simulink model "CBF_for_DoubleInteg"  (R2024a)
settings: Solver=VariableStepAuto  StartTime=0.0  StopTime=Tf  RelTol=1e-3
undefined symbols (not defined in the file): M, Ts, x1_0, x2_0
libraries: slctrl_constraint x1
settings Model: Creator=bumyong  LastModifiedBy=bumyong

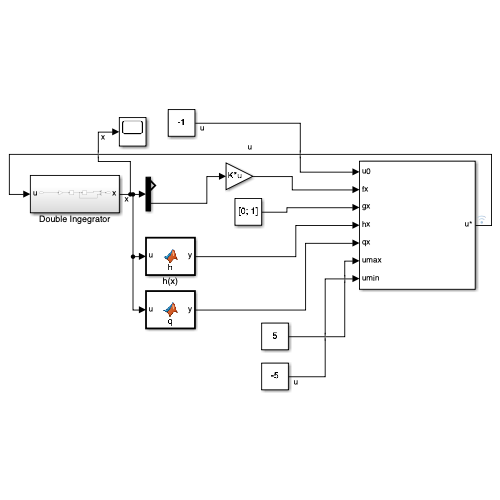
[thumbnail: Simulink's stored preview of the top-level diagram]
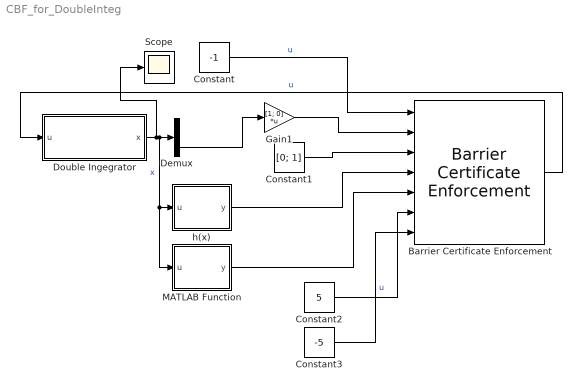
== system CBF_for_DoubleInteg ==
  Barrier Certificate Enforcement : slctrl_constraint/Barrier Certificate Enforcement  nx=2  nu=1  nc=4  gamma=gamma  beta=1  external_umax=on  external_umin=on  Ts=Ts  maxiter=200  tol=1e-6  output_exitflag=on
      settings: LibrarySourceBlock=slctrlblks/Constraint Control/Barrier Certificate Enforcement
  Constant : Constant  Value=-1
  Constant1 : Constant  Value=[0; 1]
  Constant2 : Constant  Value=5
  Constant3 : Constant  Value=-5
  Demux : Demux  Outputs=2
  Double Ingegrator : Subsystem
  Gain1 : Gain  Gain=[1; 0]  Multiplication=Matrix(K*u)
  MATLAB Function : MATLAB Function  TreatAsAtomicUnit=on
  Scope : Scope
  h(x) : MATLAB Function  TreatAsAtomicUnit=on
  wires:
  Constant/1 -> Barrier Certificate Enforcement/1  "u"
  Barrier Certificate Enforcement/1 -> Double Ingegrator/1(u)  "u"
  Constant1/1 -> Barrier Certificate Enforcement/3
  Double Ingegrator/1(x) -> Scope/1, MATLAB Function/1(u), h(x)/1(u), Demux/1  "x"
  Demux/2 -> Gain1/1
  Gain1/1 -> Barrier Certificate Enforcement/2
  h(x)/1(y) -> Barrier Certificate Enforcement/4
  MATLAB Function/1(y) -> Barrier Certificate Enforcement/5
  Constant2/1 -> Barrier Certificate Enforcement/6
  Constant3/1 -> Barrier Certificate Enforcement/7  "u"

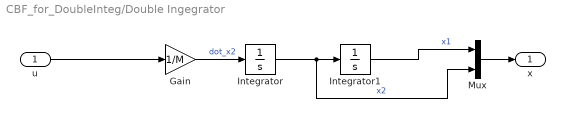
== system CBF_for_DoubleInteg/Double Ingegrator ==
  u : Inport
  Gain : Gain  Gain=1/M
  Integrator : Integrator  InitialCondition=x2_0
  Integrator1 : Integrator  InitialCondition=x1_0
  Mux : Mux  Inputs=2
  x : Outport
  wires:
  Gain/1 -> Integrator/1  "dot_x2"
  Integrator/1 -> Mux/2, Integrator1/1  "x2"
  u/1 -> Gain/1
  Integrator1/1 -> Mux/1  "x1"
  Mux/1 -> x/1

== matlab function CBF_for_DoubleInteg/h(x) ==
  data: u input; y output
function y = h(u)

    x1 = u(1);
    x2 = u(2);

    P_M = 1;
    P_m = -1;
    V_M = 1;
    V_m = -1;
    u_M = 5;
    u_m = -5;

    if x2 > 0
        h1 = P_M - x1 + x2^2/(2*u_m);
        h2 = x1 - P_m;
    else
        h1 = P_M - x1;
        h2 = x1 - P_m - x2^2/(2*u_M);
    end

    h3 = V_M - x2;
    h4 = x2 - V_m;

y = [h1; h2; h3; h4];

== matlab function CBF_for_DoubleInteg/MATLAB Function ==
  data: u input; y output
function y = q(u)
    
x1 = u(1);
x2 = u(2);

u_M = 5;
u_m = -5;

if x2 > 0
    q = [-1 x2/u_m; 1 0; 0 -1; 0 1];
else
    q = [-1 0; 1 -x2/u_M; 0 -1; 0 1];
end

y = q;
